simulink model "Simulink_Model"  (R2022a)
settings: Solver=VariableStepAuto  StartTime=0.0  StopTime=15*3600  RelTol=1e-3
PreLoadFcn:
  | % Set physical parameters
  | panelMotorParams;
values from neighbouring files (symbols this model uses):
  Damping_Constant = 8    [system_parameters.mat]
  EMF_Constant = 0.07    [system_parameters.mat]
  Gear_Ratio = 1500    [system_parameters.mat]
  Inductance = 2e-05    [system_parameters.mat]
  Inertia = 26.63    [system_parameters.mat]
  Resistence = 12    [system_parameters.mat]
  Torque_Constant = 0.07    [system_parameters.mat]
libraries: slpidlib x1
settings Model: Creator=bneiswan  LastModifiedBy=jamesbond
settings SolverCC: AlgebraicLoopSolver=TrustRegion
settings DataIOCC: ExternalInput=[sunTime sunPosition]  LoadExternalInput=on
settings DebuggingCC: UnconnectedInputMsg=warning  UnconnectedOutputMsg=warning  UnconnectedLineMsg=warning  SFMachineParentedDataDiag=warning

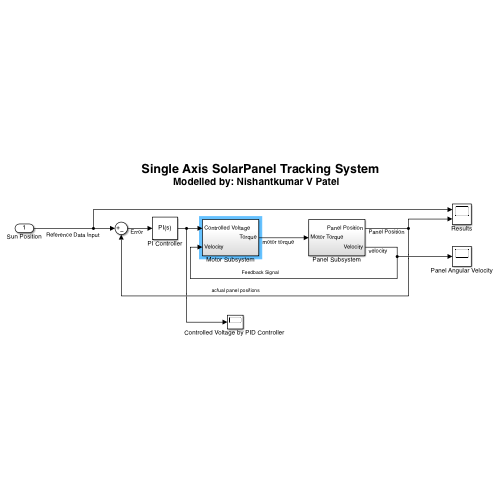
[thumbnail: Simulink's stored preview of the top-level diagram]
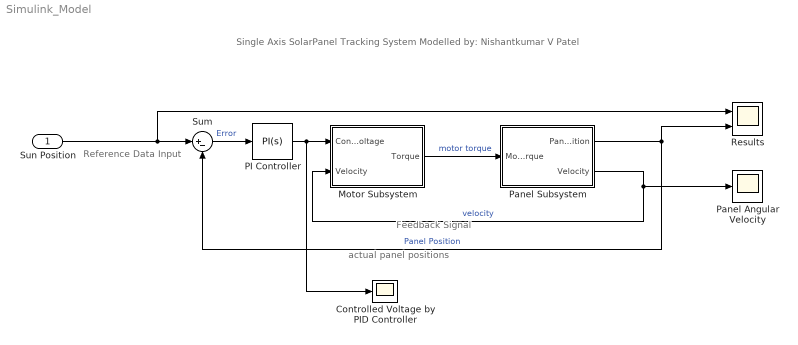
== system Simulink_Model ==
  note: Single Axis SolarPanel Tracking System
      | Modelled by: Nishantkumar V Patel
  note: Feedback Signal
  note: actual panel positions
  note: Reference Data Input
  Sun Position : Inport
  "Controlled Voltage by PID Controller " : Scope
  Motor Subsystem : Subsystem
  PI Controller : slpidlib/PID Controller  Controller=PI  Form=Parallel  TimeDomain=Continuous-time  UseExternalTs=off  SampleTime=-1  IntegratorMethod=Forward Euler  FilterMethod=Forward Euler  ControllerParametersSource=internal  P=200  I=150  UseKiTs=off  D=0  N=100  UseFilter=on  TunerSelectOption=Transfer Function Based (PID Tuner App)  InitialConditionSource=internal  InitialConditionForIntegrator=0  InitialConditionForFilter=0  DifferentiatorICPrevScaledInput=0  ExternalReset=none  TrackingMode=off  Kt=1  LimitOutput=off  SatLimitsSource=internal  UpperSaturationLimit=inf  LowerSaturationLimit=-inf  LinearizeAsGain=on  AntiWindupMode=none  Kb=1  POutMin=[]  POutMax=[]  IOutMin=[]  IOutMax=[]  DOutMin=[]  DOutMax=[]  NOutMin=[]  NOutMax=[]  SumOutMin=[]  SumOutMax=[]  SaturationOutMin=[]  SaturationOutMax=[]  PParamMin=[]  PParamMax=[]  IParamMin=[]  IParamMax=[]  DParamMin=[]  DParamMax=[]  NParamMin=[]  NParamMax=[]  KbParamMin=[]  KbParamMax=[]  KtParamMin=[]  KtParamMax=[]  KbOutMin=[]  KbOutMax=[]  KtOutMin=[]  KtOutMax=[]  IntegratorOutMin=[]  IntegratorOutMax=[]  FilterOutMin=[]  FilterOutMax=[]  SumI1OutMin=[]  SumI1OutMax=[]  SumI2OutMin=[]  SumI2OutMax=[]  SumI3OutMin=[]  SumI3OutMax=[]  SumI4OutMin=[]  SumI4OutMax=[]  SumDOutMin=[]  SumDOutMax=[]  DifferentiatorOutMin=[]  DifferentiatorOutMax=[]  FilterDiffOutCoefMin=[]  FilterDiffOutCoefMax=[]  ReciprocalOutMin=[]  ReciprocalOutMax=[]  SumDenOutMin=[]  SumDenOutMax=[]  SumNumOutMin=[]  SumNumOutMax=[]  DivideOutMin=[]  DivideOutMax=[]  UdiffTsProdOutMin=[]  UdiffTsProdOutMax=[]  NTsProdOutMin=[]  NTsProdOutMax=[]  UintegralTsProdOutMin=[]  UintegralTsProdOutMax=[]  UngainTsProdOutMin=[]  UngainTsProdOutMax=[]  IntegratorContinuousStateAttributes=''  IntegratorStateMustResolveToSignalObject=off  IntegratorRTWStateStorageClass=Auto  FilterContinuousStateAttributes=''  FilterStateMustResolveToSignalObject=off  FilterRTWStateStorageClass=Auto  ParallelPVariant=InternalParameters  IdealPVariant=Disabled  IVariant=InternalParameters  DVariant=Disabled  IntegratorVariant=Continuous  SatVariant=Disabled  AWVariant=Passthrough  PCopyVariant=Disabled  TRVariant=Disabled  FdbkBlocksVariant=Forward  IdealPFdbkVariant=Disabled  SatFdbkVariant=Disabled  DerivativeFilterVariant=Disabled  NVariant=Disabled  NCopyVariant=Disabled_SignalSpec  FilterICVariant=Disabled  IntegratorICVariant=InternalICs  ExternalResetVariant=Disabled  TRSumVariant=Passthrough  SumFdbkVariant=Disabled  SumVariant=Sum_PI  TsampFilterVariant=InternalTs  TsampNgainVariant=Passthrough  TsampIntegralVariant=Passthrough  ExternalSaturationOutDataTypeStr=Inherit: Same as second input  aMode=0
  Panel Angular Velocity : Scope
  Panel Subsystem : Subsystem
  Results : Scope  NumInputPorts=2
  Sum : Sum  Inputs=|+-
  wires:
  Panel Subsystem/1(Panel Position) -> Results/2, Sum/2  "Panel Position"
  Sum/1 -> PI Controller/1  "Error"
  Sun Position/1 -> Sum/1, Results/1
  Panel Subsystem/2(Velocity) -> Motor Subsystem/2(Velocity), Panel Angular Velocity/1  "velocity"
  PI Controller/1 -> Motor Subsystem/1(Controlled Voltage), "Controlled Voltage by PID Controller "/1
  Motor Subsystem/1(Torque) -> Panel Subsystem/1(Motor Torque)  "motor torque"

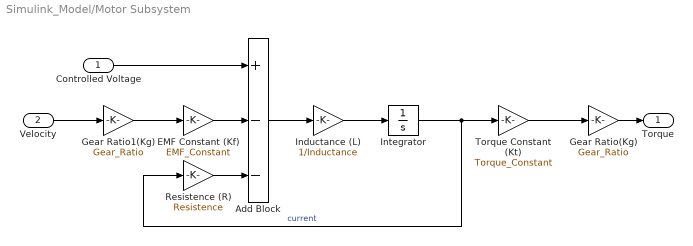
== system Simulink_Model/Motor Subsystem ==
  Controlled Voltage : Inport
  Velocity : Inport  Port=2
  Add Block : Sum  Inputs=+--
  EMF Constant (Kf) : Gain  Gain=EMF_Constant
  Gear Ratio(Kg) : Gain  Gain=Gear_Ratio
  "Gear Ratio1(Kg)  " : Gain  Gain=Gear_Ratio
  Inductance (L) : Gain  Gain=1/Inductance
  Integrator : Integrator
  Resistence (R) : Gain  Gain=Resistence
  "Torque Constant (Kt) " : Gain  Gain=Torque_Constant
  Torque : Outport
  wires:
  Controlled Voltage/1 -> Add Block/1
  EMF Constant (Kf)/1 -> Add Block/2
  Inductance (L)/1 -> Integrator/1
  Resistence (R)/1 -> Add Block/3
  Integrator/1 -> "Torque Constant (Kt) "/1, Resistence (R)/1  "current"
  Add Block/1 -> Inductance (L)/1
  Velocity/1 -> "Gear Ratio1(Kg)  "/1
  "Torque Constant (Kt) "/1 -> Gear Ratio(Kg)/1
  "Gear Ratio1(Kg)  "/1 -> EMF Constant (Kf)/1
  Gear Ratio(Kg)/1 -> Torque/1

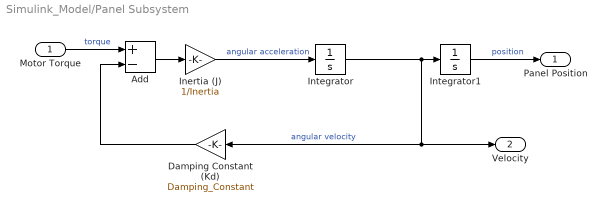
== system Simulink_Model/Panel Subsystem ==
  Motor Torque : Inport
  Add : Sum  Inputs=+-
  Damping Constant (Kd) : Gain  Gain=Damping_Constant
  Inertia (J) : Gain  Gain=1/Inertia
  Integrator : Integrator
  Integrator1 : Integrator
  Panel Position : Outport
  Velocity : Outport  Port=2
  wires:
  Motor Torque/1 -> Add/1  "torque"
  Add/1 -> Inertia (J)/1
  Integrator/1 -> Integrator1/1, Damping Constant (Kd)/1, Velocity/1  "angular velocity"
  Damping Constant (Kd)/1 -> Add/2
  Inertia (J)/1 -> Integrator/1  "angular acceleration"
  Integrator1/1 -> Panel Position/1  "position"
